simulink model "auto_climate_elec"  (Simulink 6.0)
settings: Solver=ode23tb  StartTime=0.0  StopTime=inf  RelTol=1e-3
libraries: powerlib2 x12, simulink x2, simulink_extras x2, powerlib_extras x1
settings Model: Creator=The MathWorks Inc.  LastModifiedBy=batserve  ExtModeAutoUpdateStatusClock=off
settings DataIOCC: SignalLoggingName=sigsOut
settings OptimizationCC: BooleanDataType=off
settings DebuggingCC: CheckExecutionContextPreStartOutputMsg=on  CheckExecutionContextRuntimeOutputMsg=on  SolverPrmCheckMsg=none
settings HardwareCC: TargetUnknown=on

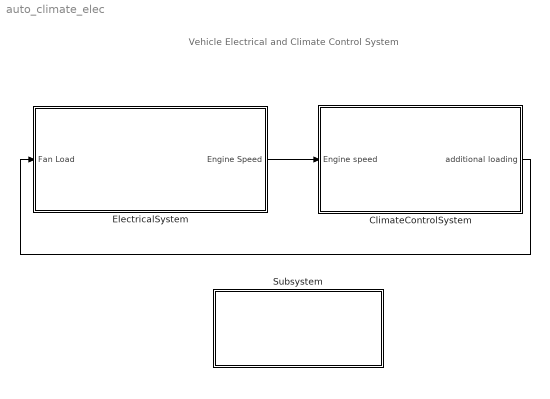
== system auto_climate_elec ==
  note: Vehicle Electrical and Climate Control System
  ClimateControlSystem : Subsystem  PropExecContextAcrossSSBoundary=on
  ElectricalSystem : Subsystem  PropExecContextAcrossSSBoundary=on
  Subsystem : Subsystem  Orientation=down  PropExecContextAcrossSSBoundary=on
      mask init:
      | %t=matlabroot;
      | %cd(t)
      | %test123=which('doc_file.html','-all');
      | %web(char(test123));
      settings: AttributesFormatString=\n
      settings: OpenFcn=|
      | docfile=which('auto_climate_elec.html','-all');
      | web(char(docfile));
      mask Display: disp('Double click\nhere for\n Model Information')
  wires:
  ElectricalSystem/1(Engine Speed) -> ClimateControlSystem/1(Engine speed)
  ClimateControlSystem/1(additional loading) -> ElectricalSystem/1(Fan Load)

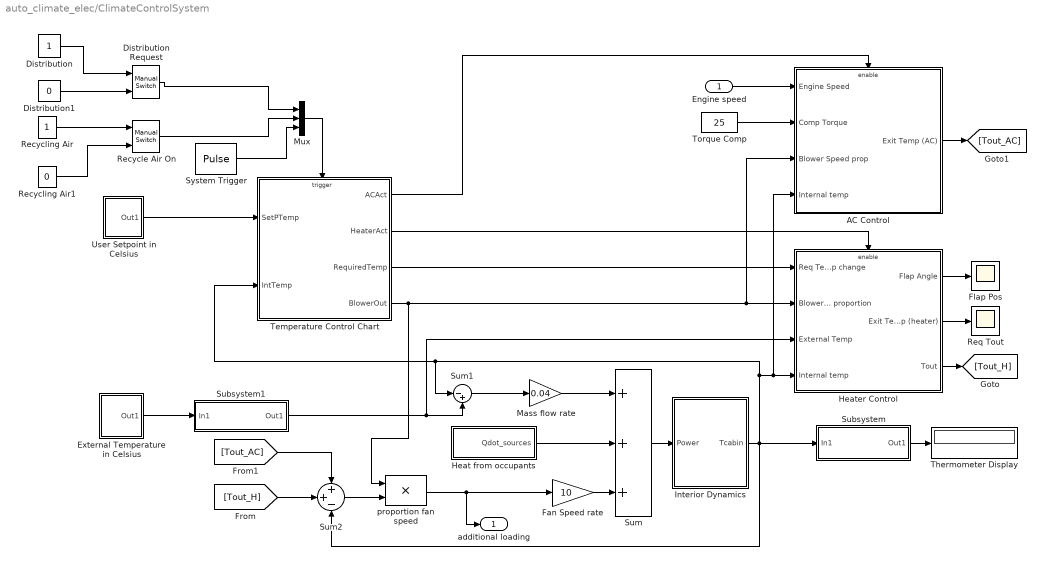
== system auto_climate_elec/ClimateControlSystem ==
  Engine speed : Inport  Port=1  LatchInput=off
  AC Control : Subsystem  TreatAsAtomicUnit=on  PropExecContextAcrossSSBoundary=on
  "Distribution " : Constant
  Distribution Request : simulink/Signal Routing/Manual Switch  sw=0  action=0
  "Distribution1 " : Constant  Value=0
  External Temperature in Celsius : Subsystem  PropExecContextAcrossSSBoundary=on  mask(variable){x=18}
      mask prompts: x "Enter the external temperature"
      mask init:
      | set_param('auto_climate_elec/ClimateControlSystem/External Temperature in Celsius/External Temp','Value',num2str(x))
      | external_temp_limit
      mask Display: disp(x);
  Fan Speed rate : Gain  Gain=10  SaturateOnIntegerOverflow=on
  Flap Pos : Scope
      settings: YMin=41.175  YMax=41.22
  Heat from occupants : Subsystem  PropExecContextAcrossSSBoundary=on  mask(Heat from occupants){N=1}
      mask prompts: N "Number of occupants:"
      settings: AttributesFormatString=No. of occupants: %<N>
      mask Display: disp('Heat Sources')
  Heater Control : Subsystem  TreatAsAtomicUnit=on  PropExecContextAcrossSSBoundary=on
  Interior Dynamics : Subsystem  PropExecContextAcrossSSBoundary=on
      mask Type: Vehicle Cabin Dynamics
      mask Display: image(imread('car_int.jpg'))
  Mass flow rate : Gain  Gain=0.04  SaturateOnIntegerOverflow=on
  Mux : Mux  Inputs=3
  Recycle Air On : simulink/Signal Routing/Manual Switch  sw=0  action=0
  Recycling Air : Constant
  Recycling Air1 : Constant  Value=0
  Req Tout : Scope
      settings: YMin=41.175  YMax=41.22
  Subsystem : Subsystem  PropExecContextAcrossSSBoundary=on
      mask Display: disp('Kelvin to Celsius')
  Subsystem1 : Subsystem  PropExecContextAcrossSSBoundary=on
      mask Display: disp('Celsius to Kelvin')
  Sum : Sum  Inputs=+++  SaturateOnIntegerOverflow=on  InputSameDT=on
  Sum1 : Sum  Inputs=|-+  SaturateOnIntegerOverflow=on  InputSameDT=on
  Sum2 : Sum  Inputs=++-  SaturateOnIntegerOverflow=on  InputSameDT=on
  System Trigger : DiscretePulseGenerator  PulseType=Time based  Period=1/60  PulseWidth=50
  Temperature Control Chart : Stateflow chart  TreatAsAtomicUnit=on  PropExecContextAcrossSSBoundary=on
  Thermometer Display : Display
  Torque Comp : Constant  Value=25
  User Setpoint in Celsius : Subsystem  PropExecContextAcrossSSBoundary=on  mask{USet=9}
      mask prompts: USet "Enter the Temperature you require"
      mask init:
      | set_param('auto_climate_elec/ClimateControlSystem/User Setpoint in Celsius/User Setpoint','Value',num2str(USet))
      mask Display: disp(num2str(USet))
  proportion fan speed : Product  SaturateOnIntegerOverflow=on  InputSameDT=on
  additional loading : Outport
  wires:
  Distribution Request/1 -> Mux/1
  "Distribution "/1 -> Distribution Request/1
  "Distribution1 "/1 -> Distribution Request/2
  Recycling Air1/1 -> Recycle Air On/2
  User Setpoint in Celsius/1(Out1) -> Temperature Control Chart/1(SetPTemp)
  Recycling Air/1 -> Recycle Air On/1
  Recycle Air On/1 -> Mux/2
  System Trigger/1 -> Mux/3
  Interior Dynamics/1("Tcabin ") -> AC Control/4(Internal temp), Heater Control/4(Internal temp), Temperature Control Chart/2(IntTemp), Sum1/1, Sum2/3, Subsystem/1(In1)
  Subsystem/1(Out1) -> Thermometer Display/1
  Heat from occupants/1(Qdot_sources) -> Sum/2
  External Temperature in Celsius/1(Out1) -> Subsystem1/1(In1)
  Mass flow rate/1 -> Sum/1
  Sum1/1 -> Mass flow rate/1
  Subsystem1/1(Out1) -> Heater Control/3(External Temp), Sum1/2
  Fan Speed rate/1 -> Sum/3
  Sum2/1 -> proportion fan speed/2
  Temperature Control Chart/4(BlowerOut) -> AC Control/3(Blower Speed prop), Heater Control/2(Blower Speed proportion), proportion fan speed/1
  proportion fan speed/1 -> additional loading/1, Fan Speed rate/1
  Temperature Control Chart/2(HeaterAct) -> Heater Control/Enable
  Heater Control/1(Flap Angle) -> Flap Pos/1
  Heater Control/2(Exit Temp (heater)) -> Req Tout/1
  Heater Control/3(Tout) -> [Tout_H]
  [Tout_H] -> Sum2/2
  Temperature Control Chart/1(ACAct) -> AC Control/Enable
  [Tout_AC] -> Sum2/1
  Torque Comp/1 -> AC Control/2(Comp Torque)
  Temperature Control Chart/3(RequiredTemp) -> Heater Control/1(Req Temp change)
  AC Control/1(Exit Temp (AC)) -> [Tout_AC]
  Engine speed/1 -> AC Control/1(Engine Speed)
  Mux/1 -> Temperature Control Chart/Trigger
  Sum/1 -> Interior Dynamics/1(Power)

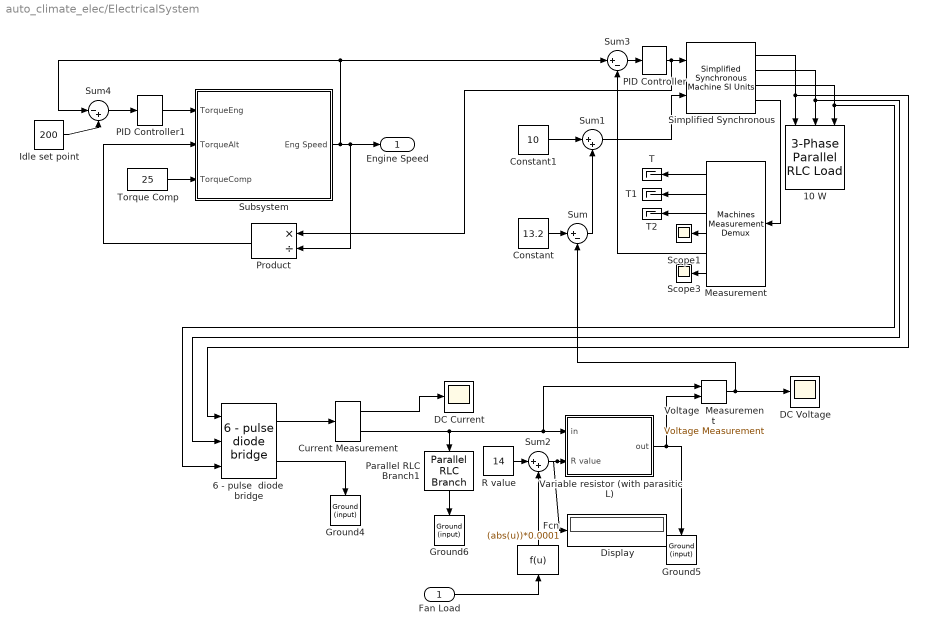
== system auto_climate_elec/ElectricalSystem ==
  Fan Load : Inport  Port=1  LatchInput=off
  " DC Current" : Scope
      settings: YMin=15  YMax=16.75
  10 W : powerlib2/Elements/3-Phase Parallel RLC Load  Orientation=down  Vpp=20  fn=60  P3=1  QL3=0  QC3=0
  6 - pulse  diode  bridge : powerlib_extras/Three-Phase Library/6 - pulse  diode  bridge  Ron=0.01  Lon=10e-6  Vf=0.8  Rs=1e10  Cs=100e-09
  Constant : Constant  Value=13.2
  Constant1 : Constant  Value=10
  Current Measurement : powerlib2/Measurements/Current Measurement  Tag=PoWeRsYsTeMmEaSuReMeNt  PhasorSimulation=off  OutputType=Magnitude  PSBOutputType=01  PSBequivalent=0
  DC Voltage : Scope
      settings: YMin=11.9  YMax=12.9  SaveName=ScopeData3
  Display : Display
  Fcn : Fcn  Orientation=up  Expr=(abs(u))*0.0001
  Ground4 : powerlib2/Connectors/Ground (input)  Tag=PoWeRsYsTeMbLoCk  Orientation=down
  Ground5 : powerlib2/Connectors/Ground (input)  Tag=PoWeRsYsTeMbLoCk  Orientation=down
  Ground6 : powerlib2/Connectors/Ground (input)  Tag=PoWeRsYsTeMbLoCk  Orientation=down
  Idle set point : Constant  Value=200
  Measurement : powerlib2/Machines/Machines Measurement Demux  Orientation=left  machType=Simplified synchronous  ssm1=on  ssm2=on  ssm3=on  ssm4=on  ssm5=on  ssm6=on  sm1=on  sm2=on  sm3=on  sm4=on  sm5=on  sm6=on  sm7=on  sm8=on  sm9=on  sm10=on  sm11=on  sm115=off  sm12=off  sm13=off  sm14=off  asm1=on  asm2=on  asm3=on  asm4=on  asm5=on  asm6=on  asm7=on  asm8=on  asm9=on  asm10=on  asm11=on  pmsm1=on  pmsm2=on  pmsm3=on  pmsm4=on  pmsm5=on  pmsm6=on  lastType=1
  PID Controller : simulink_extras/Additional Linear/PID Controller  P=2  I=8  D=1
  PID Controller1 : simulink_extras/Additional Linear/PID Controller  P=2  I=8  D=0
  Parallel RLC Branch1 : powerlib2/Elements/Parallel RLC Branch  Tag=PoWeRsYsTeMbLoCk  Orientation=down  a=100  b=inf  c=50e-06  mesure=None  PSBOutputType=1
  Product : Product  Orientation=left  Inputs=*/  SaturateOnIntegerOverflow=on  InputSameDT=on
  R value : Constant  Value=14
  Scope1 : Scope
      settings: YMin=-17.5  YMax=17.5  SaveName=ScopeData2
  Scope3 : Scope
      settings: YMin=-17.5  YMax=17.5  SaveName=ScopeData4
  "Simplified Synchronous " : powerlib2/Machines/Simplified Synchronous  Machine SI Units  Tag=PoWeRsYsTeMbLoCk  conType=3-wire Y  x1=[ 750, 20, 60 ]  x2=[ inf, 0, 3]  x3=[ 0.1, 2.15e-5 ]  x4="[ 0   0   0,0,0   0,0,0 ]"  PSBOutputType=1111  iounits=1  LoadFlowParameters=[1,0,0,0,0]
  Subsystem : Subsystem  PropExecContextAcrossSSBoundary=on
  Sum : Sum  Inputs=|+-  SaturateOnIntegerOverflow=on  InputSameDT=on
  Sum1 : Sum  Inputs=|++  SaturateOnIntegerOverflow=on  InputSameDT=on
  Sum2 : Sum  Inputs=|++  SaturateOnIntegerOverflow=on  InputSameDT=on
  Sum3 : Sum  Inputs=|+-  SaturateOnIntegerOverflow=on  InputSameDT=on
  Sum4 : Sum  Inputs=|-+  SaturateOnIntegerOverflow=on  InputSameDT=on
  T : Terminator
  T1 : Terminator
  T2 : Terminator
  Torque Comp : Constant  Value=25
  "Variable resistor (with parasitic L) " : Subsystem  PropExecContextAcrossSSBoundary=on
      mask init:
      | [s1,s2,s3,s4,r1,r2,l1,l2,c1,c2,c3,c4,x1,x2,x3,x4] = powericon('Parallel RLC Branch',1,inf,0);
      mask Display: plot(s1-30,s2,s3+30,s4,r1,r2,l1,l2,c1,c2,c3,c4,x1,x2,x3,x4)
  Voltage  Measurement : powerlib2/Measurements/Voltage Measurement  Tag=PoWeRsYsTeMmEaSuReMeNt  PhasorSimulation=off  OutputType=Magnitude  PSBOutputType=0  PSBequivalent=1
  Engine Speed : Outport  InitialOutput=0
  wires:
  "Simplified Synchronous "/2 -> 10 W/2, 6 - pulse  diode  bridge/2
  "Simplified Synchronous "/1 -> 10 W/1, 6 - pulse  diode  bridge/1
  "Simplified Synchronous "/3 -> 10 W/3, 6 - pulse  diode  bridge/3
  6 - pulse  diode  bridge/2 -> Ground4/1
  Parallel RLC Branch1/1 -> Ground6/1
  Constant1/1 -> Sum1/1
  Sum/1 -> Sum1/2
  Sum1/1 -> "Simplified Synchronous "/2
  Voltage  Measurement/1 -> DC Voltage/1, Sum/2
  6 - pulse  diode  bridge/1 -> Current Measurement/1
  Current Measurement/2 -> Parallel RLC Branch1/1, "Variable resistor (with parasitic L) "/1(in), Voltage  Measurement/1
  Current Measurement/1 -> " DC Current"/1
  "Variable resistor (with parasitic L) "/1(out) -> Ground5/1, Voltage  Measurement/2
  Sum2/1 -> "Variable resistor (with parasitic L) "/2(R value), Display/1
  R value/1 -> Sum2/1
  Fan Load/1 -> Fcn/1
  Subsystem/1(Eng Speed) -> Sum3/1, Sum4/1, Product/2, Engine Speed/1
  Torque Comp/1 -> Subsystem/3(TorqueComp)
  Constant/1 -> Sum/1
  "Simplified Synchronous "/4 -> Measurement/1
  Measurement/1 -> T/1
  Measurement/2 -> T1/1
  Measurement/3 -> T2/1
  Measurement/4 -> Scope1/1
  Measurement/6 -> Scope3/1
  Sum3/1 -> PID Controller/1
  Measurement/5 -> Sum3/2
  Sum4/1 -> PID Controller1/1
  Idle set point/1 -> Sum4/2
  PID Controller/1 -> "Simplified Synchronous "/1, Product/1
  PID Controller1/1 -> Subsystem/1(TorqueEng)
  Product/1 -> Subsystem/2(TorqueAlt)
  Fcn/1 -> Sum2/2

== system auto_climate_elec/Subsystem ==

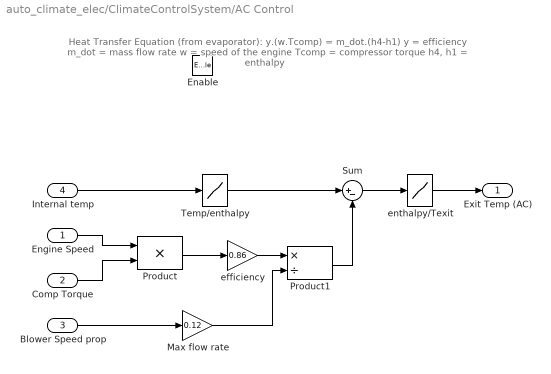
== system auto_climate_elec/ClimateControlSystem/AC Control ==
  note: Heat Transfer Equation (from evaporator):
      |
      | y.(w.Tcomp) = m_dot.(h4-h1)
      |
      | y = efficiency
      | m_dot = mass flow rate
      | w = speed of the engine
      | Tcomp = compressor torque
      | h4, h1 = enthalpy
  Engine Speed : Inport  Port=1  LatchInput=off
  Comp Torque : Inport  Port=2  LatchInput=off
  Blower Speed prop : Inport  Port=3  LatchInput=off
  Internal temp : Inport  Port=4  LatchInput=off
  Enable : EnablePort  StatesWhenEnabling=reset  ZeroCross=off
  Max flow rate : Gain  Gain=0.12  SaturateOnIntegerOverflow=on
  Product : Product  SaturateOnIntegerOverflow=on  InputSameDT=on
  Product1 : Product  Inputs=*/  SaturateOnIntegerOverflow=on  InputSameDT=on
  Sum : Sum  Inputs=|+-  SaturateOnIntegerOverflow=on  InputSameDT=on
  Temp/enthalpy : Lookup  DialogController=Simulink.DDGSource  InputValues=[220 230 240 250 260 270 280 285 290 295 300 305 310 315 320]  OutputValues=[219.97 230.02 240.02 250.05 260.09 270.11 280.13 285.14 290.16 295.17 300.19 305.22 310.24 315.27 320.29]  SaturateOnIntegerOverflow=on
  efficiency : Gain  Gain=0.86  SaturateOnIntegerOverflow=on
  enthalpy/Texit : Lookup  DialogController=Simulink.DDGSource  InputValues=[219.97 230.02 240.02 250.05 260.09 270.11 280.13 285.14 290.16 295.17 300.19 305.22 310.24 315.27 320.29]  OutputValues=[220 230 240 250 260 270 280 285 290 295 300 305 310 315 320]  SaturateOnIntegerOverflow=on
  Exit Temp (AC) : Outport  OutputWhenDisabled=reset  InitialOutput=0
  wires:
  Sum/1 -> enthalpy/Texit/1
  Product1/1 -> Sum/2
  Temp/enthalpy/1 -> Sum/1
  Internal temp/1 -> Temp/enthalpy/1
  enthalpy/Texit/1 -> Exit Temp (AC)/1
  Max flow rate/1 -> Product1/2
  Blower Speed prop/1 -> Max flow rate/1
  efficiency/1 -> Product1/1
  Product/1 -> efficiency/1
  Comp Torque/1 -> Product/2
  Engine Speed/1 -> Product/1

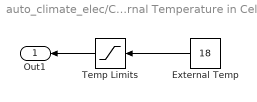
== system auto_climate_elec/ClimateControlSystem/External Temperature in Celsius ==
  External Temp : Constant  Orientation=left  Value=18
  Temp Limits : Saturate  Orientation=left  UpperLimit=100  LowerLimit=-99
  Out1 : Outport  Orientation=left
  wires:
  External Temp/1 -> Temp Limits/1
  Temp Limits/1 -> Out1/1

== system auto_climate_elec/ClimateControlSystem/Heat from occupants ==
  No of occupants : Gain  Gain=N  SaturateOnIntegerOverflow=on
  Power per occupant [W] : Constant  Value=100
  Qdot_sources : Outport
  wires:
  Power per occupant [W]/1 -> No of occupants/1
  No of occupants/1 -> Qdot_sources/1  "Qdot_sources"

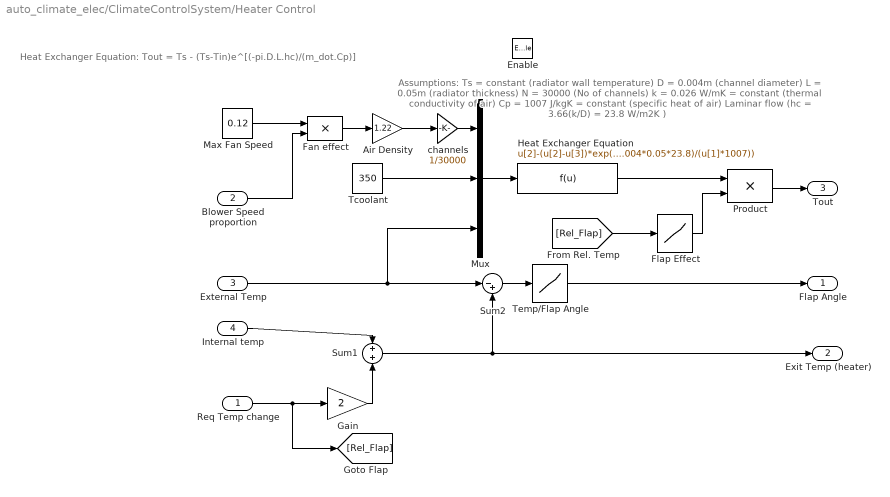
== system auto_climate_elec/ClimateControlSystem/Heater Control ==
  note: Assumptions:
      | Ts = constant (radiator wall temperature)
      | D = 0.004m (channel diameter)
      | L = 0.05m (radiator thickness)
      | N = 30000 (No of channels)
      |
      | k = 0.026 W/mK = constant (thermal conductivity of air)
      | Cp = 1007 J/kgK = constant (specific heat of air)
      | Laminar flow (hc = 3.66(k/D) = 23.8 W/m2K )
  note: Heat Exchanger Equation:
      | Tout = Ts - (Ts-Tin)e^[(-pi.D.L.hc)/(m_dot.Cp)]
  Req Temp change : Inport  Port=1  LatchInput=off
  Blower Speed proportion : Inport  Port=2  LatchInput=off
  External Temp : Inport  Port=3  LatchInput=off
  Internal temp : Inport  Port=4  LatchInput=off
  Enable : EnablePort  StatesWhenEnabling=reset  ZeroCross=off
  Air Density : Gain  Gain=1.22  SaturateOnIntegerOverflow=on
  Fan effect : Product  SaturateOnIntegerOverflow=on  InputSameDT=on
  Flap Effect : Lookup  DialogController=Simulink.DDGSource  InputValues="[0 3 5 10 50  90 100 200 ]"  OutputValues="[0 300 100  10 10  10 3 1]"  SaturateOnIntegerOverflow=on
  Gain : Gain  Gain=2  SaturateOnIntegerOverflow=on
  Heat Exchanger Equation : Fcn  Expr=u[2]-(u[2]-u[3])*exp(-(pi*0.004*0.05*23.8)/(u[1]*1007))
  Max Fan Speed : Constant  Value=0.12
  Mux : Mux  Inputs=3
  Product : Product  SaturateOnIntegerOverflow=on  InputSameDT=on
  Sum1 : Sum  SaturateOnIntegerOverflow=on  InputSameDT=on
  Sum2 : Sum  Inputs=|-+  SaturateOnIntegerOverflow=on  InputSameDT=on
  "Tcoolant " : Constant  Value=350
  Temp/Flap Angle : Lookup  DialogController=Simulink.DDGSource  InputValues=[0 10 20 30 40 50 60 75 100 200]  OutputValues=[0 20 30 45 60 75 90 90 90 90]  SaturateOnIntegerOverflow=on
  channels : Gain  Gain=1/30000  SaturateOnIntegerOverflow=on
  Flap Angle : Outport  OutputWhenDisabled=reset  InitialOutput=0
  Exit Temp (heater) : Outport  Port=2  OutputWhenDisabled=reset  InitialOutput=0
  Tout : Outport  Port=3  OutputWhenDisabled=reset  InitialOutput=0
  wires:
  Heat Exchanger Equation/1 -> Product/1
  External Temp/1 -> Mux/3, Sum2/1
  Blower Speed proportion/1 -> Fan effect/2
  Max Fan Speed/1 -> Fan effect/1
  Fan effect/1 -> Air Density/1
  Mux/1 -> Heat Exchanger Equation/1
  Air Density/1 -> channels/1
  channels/1 -> Mux/1
  "Tcoolant "/1 -> Mux/2
  Product/1 -> Tout/1
  Temp/Flap Angle/1 -> Flap Angle/1
  Sum2/1 -> Temp/Flap Angle/1
  Internal temp/1 -> Sum1/1
  Gain/1 -> Sum1/2
  Sum1/1 -> Exit Temp (heater)/1, Sum2/2
  Req Temp change/1 -> Gain/1, [Rel_Flap]
  Flap Effect/1 -> Product/2
  [Rel_Flap] -> Flap Effect/1

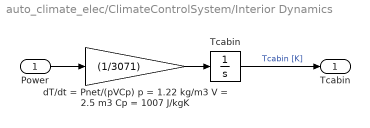
== system auto_climate_elec/ClimateControlSystem/Interior Dynamics ==
  Power : Inport  Port=1  LatchInput=off
  Tcabin : Integrator  InitialCondition=291  ZeroCross=off
  dT/dt = Pnet/(pVCp) p = 1.22 kg/m3 V = 2.5 m3 Cp = 1007 J/kgK : Gain  Gain=(1/3071)  SaturateOnIntegerOverflow=on
  "Tcabin " : Outport
  wires:
  dT/dt = Pnet/(pVCp) p = 1.22 kg/m3 V = 2.5 m3 Cp = 1007 J/kgK/1 -> Tcabin/1
  Power/1 -> dT/dt = Pnet/(pVCp) p = 1.22 kg/m3 V = 2.5 m3 Cp = 1007 J/kgK/1
  Tcabin/1 -> "Tcabin "/1  "Tcabin [K]"

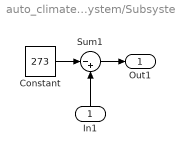
== system auto_climate_elec/ClimateControlSystem/Subsystem ==
  In1 : Inport  Orientation=up  Port=1  LatchInput=off
  Constant : Constant  Value=273
  Sum1 : Sum  Inputs=|-+  SaturateOnIntegerOverflow=on  InputSameDT=on
  Out1 : Outport
  wires:
  Sum1/1 -> Out1/1
  In1/1 -> Sum1/2
  Constant/1 -> Sum1/1

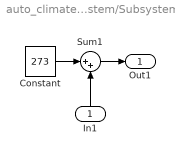
== system auto_climate_elec/ClimateControlSystem/Subsystem1 ==
  In1 : Inport  Orientation=up  Port=1  LatchInput=off
  Constant : Constant  Value=273
  Sum1 : Sum  Inputs=|++  SaturateOnIntegerOverflow=on  InputSameDT=on
  Out1 : Outport
  wires:
  Constant/1 -> Sum1/1
  In1/1 -> Sum1/2
  Sum1/1 -> Out1/1

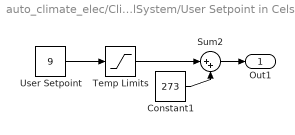
== system auto_climate_elec/ClimateControlSystem/User Setpoint in Celsius ==
  Constant1 : Constant  Value=273
  Sum2 : Sum  Inputs=|++  SaturateOnIntegerOverflow=on  InputSameDT=on
  Temp Limits : Saturate  UpperLimit=100  LowerLimit=-99
  User Setpoint : Constant  Value=9
  Out1 : Outport
  wires:
  Sum2/1 -> Out1/1
  User Setpoint/1 -> Temp Limits/1
  Constant1/1 -> Sum2/2
  Temp Limits/1 -> Sum2/1

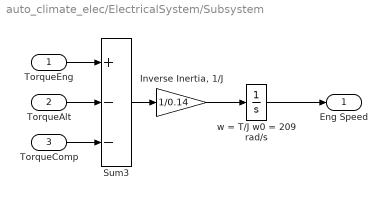
== system auto_climate_elec/ElectricalSystem/Subsystem ==
  TorqueEng : Inport  Port=1  LatchInput=off
  TorqueAlt : Inport  Port=2  LatchInput=off
  TorqueComp : Inport  Port=3  LatchInput=off
  "Inverse Inertia, 1/J" : Gain  Gain=1/0.14  SaturateOnIntegerOverflow=on
  Sum3 : Sum  Inputs=+--  SaturateOnIntegerOverflow=on  InputSameDT=on
  w = T/J w0 = 209 rad/s : Integrator  InitialCondition=209.48  ZeroCross=off
  Eng Speed : Outport  InitialOutput=0
  wires:
  "Inverse Inertia, 1/J"/1 -> w = T/J w0 = 209 rad/s/1
  w = T/J w0 = 209 rad/s/1 -> Eng Speed/1
  Sum3/1 -> "Inverse Inertia, 1/J"/1
  TorqueEng/1 -> Sum3/1
  TorqueAlt/1 -> Sum3/2
  TorqueComp/1 -> Sum3/3

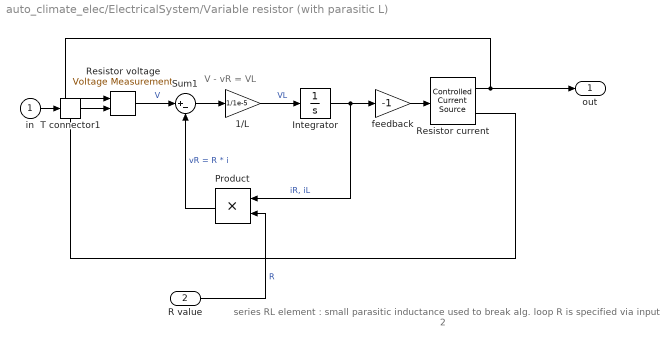
== system auto_climate_elec/ElectricalSystem/Variable resistor (with parasitic L)  ==
  note: V - vR = VL
  note: series RL element : small parasitic inductance used to break alg. loop
      | R is specified via input 2
  in : Inport  Port=1  LatchInput=off
  R value : Inport  Port=2  LatchInput=off
  1/L : Gain  Gain=1/1e-5  SaturateOnIntegerOverflow=on
  Integrator : Integrator  ZeroCross=off
  Product : Product  Orientation=left  SaturateOnIntegerOverflow=on  InputSameDT=on
  Resistor current : powerlib2/Electrical Sources/Controlled Current Source  Tag=PoWeRsYsTeMbLoCk  Description=source block  initsrc=on  srctyp=DC  ia=0  iph=0  freq=0  mesure=None  PSBOutputType=11
  Resistor voltage : powerlib2/Measurements/Voltage Measurement  Tag=PoWeRsYsTeMmEaSuReMeNt  PhasorSimulation=off  OutputType=Magnitude  PSBOutputType=0  PSBequivalent=0
  Sum1 : Sum  Inputs=|+-  SaturateOnIntegerOverflow=on  InputSameDT=on
  T connector1 : powerlib2/Connectors/T connector  Tag=PoWeRsYsTeMbLoCk  PSBOutputType=1
  feedback : Gain  Gain=-1  SaturateOnIntegerOverflow=on
  out : Outport
  wires:
  Resistor current/1 -> out/1, Resistor voltage/1
  in/1 -> T connector1/1
  Sum1/1 -> 1/L/1
  Resistor current/2 -> T connector1/Enable
  T connector1/1 -> Resistor voltage/2
  Integrator/1 -> Product/1, feedback/1  "iR, iL"
  1/L/1 -> Integrator/1  "VL"
  Resistor voltage/1 -> Sum1/1  "V"
  R value/1 -> Product/2  "R"
  Product/1 -> Sum1/2  "vR = R * i"
  feedback/1 -> Resistor current/1

== stateflow chart ClimateControlSystem/Temperature Control Chart ==
  state Blower [parallel]
    during:setpoint_calc();
    state Blower_off
      entry:BlowerOut=0.0;
    state Blower_on
      state Blower_1
        entry:BlowerOut=0.2;
      state Blower_2
        entry:BlowerOut=0.4;
      state Blower_3
        entry:BlowerOut=0.6;
      state Blower_5
        entry:BlowerOut=1.0;
      state Blower_4
        entry:BlowerOut=0.8;
      Blower_on -> Blower_2 : E[!in(Blower_2) && in_temp_range(7,10)]
      Blower_on -> Blower_1 : E[!in(Blower_1) && in_temp_range(1.5,5)]
      Blower_on -> Blower_3 : E[!in(Blower_3) && in_temp_range(12,15)]
      Blower_on -> Blower_4 : E[!in(Blower_4) && in_temp_range(17,20)]
      Blower_on -> Blower_5 : E[!in(Blower_5) && in_temp_range(22,200)]
      (default) -> Blower_1
    state b = in_temp_range(minTemp,maxTemp) [function]
      (default) -> (junction 26) : {b = (absTempDiff>minTemp) &&  ...
          |         (absTempDiff<maxTemp);}
    state setpoint_calc() [function]
      (default) -> (junction 27) : {RequiredTemp = SetPTemp-IntTemp;}
      (junction 27) -> (junction 24) : [RequiredTemp<0.0]
          | {absTempDiff = -RequiredTemp;}
      (junction 27) -> (junction 25) : {absTempDiff = RequiredTemp;}
    (default) -> Blower_off
    Blower_on -> Blower_off : E[absTempDiff>203 || absTempDiff<=0.5]
    Blower_off -> Blower_on : E[in_temp_range(.5,203)]
  state Recyc_Air [parallel]
    state Recyc_on
    state Recyc_off
    Recyc_on -> Recyc_off : en(AirDist.Defrost)
    (default) -> Recyc_on
    Recyc_on -> Recyc_off : RecycReq
    Recyc_off -> Recyc_on : RecycReq
  state Heater_AC [parallel]
    state H_offAC_off
    state HeaterAct
    state ACAct
    ACAct -> H_offAC_off : E[SetPTemp-IntTemp>=-0.5]
    H_offAC_off -> ACAct : E[SetPTemp-IntTemp<-0.5]
    H_offAC_off -> HeaterAct : E[SetPTemp-IntTemp>0.5]
    HeaterAct -> H_offAC_off : E[SetPTemp-IntTemp<=0.5]
    (default) -> H_offAC_off
  state AirDist [parallel]
    state Face
    state Feet
    state Defrost
    (default) -> Face
    Defrost -> Face : DistReq
    Feet -> Defrost : DistReq
    Face -> Feet : DistReq
  data: minTemp function_input double; b function_output boolean; maxTemp function_input double; ACAct output State; SetPTemp input double; IntTemp input double; HeaterAct output State; RequiredTemp output double; BlowerOut output double; absTempDiff local double
  events: DistReq input EITHER_EDGE_EVENT; RecycReq input EITHER_EDGE_EVENT; E input EITHER_EDGE_EVENT
